simulink model "basebot_model_sampling"  (R2026a)
settings: Solver=ode45  StopTime=0.6  MaxStep=min(Ts/10,0.001)  RelTol=1e-6  AbsTol=1e-9
model workspace (MAT data in the model file):
  D = 1e-05
  J = 1e-05
  Kb = 0.01
  Kp = 0.05
  Kt = 0.01
  L = 0.001
  R = 1
  Ts = 0.001
  gear = 9.68
  referenceSpeed = 0.1
  stepTime = 0.2
  wheelRadius = 0.03
settings Model: Creator=michaeljohansen  LastModifiedBy=michaeljohansen

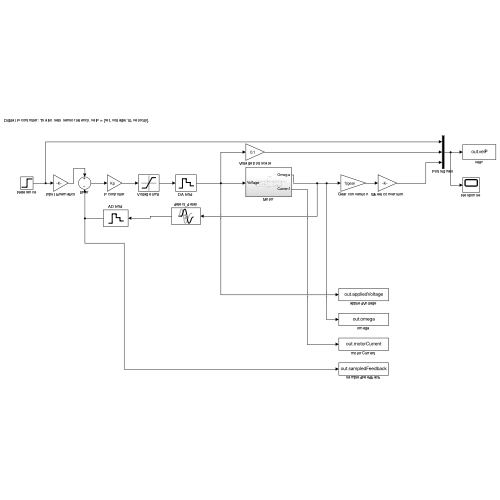
[thumbnail: Simulink's stored preview of the top-level diagram]
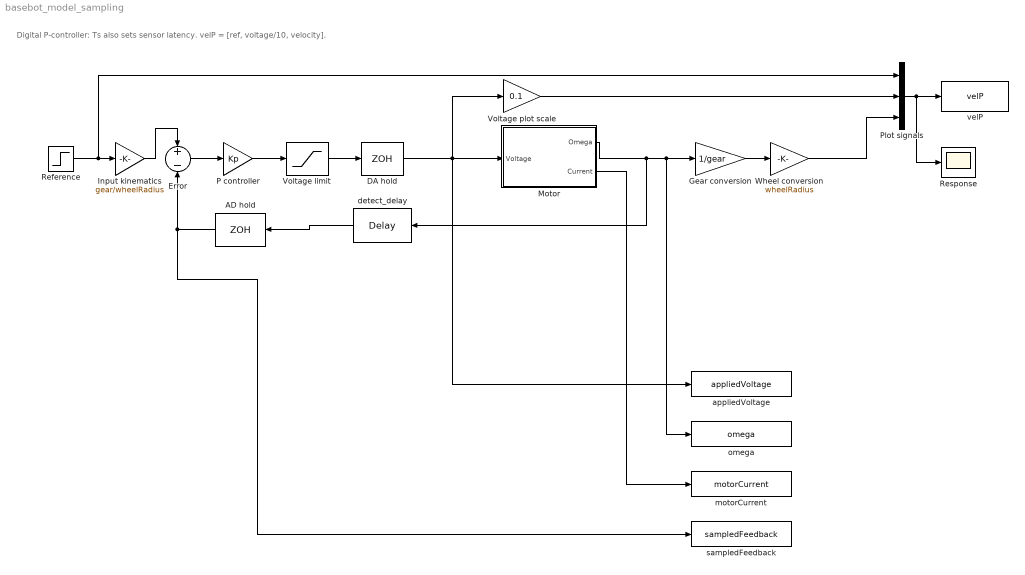
== system basebot_model_sampling ==
  note: Digital P-controller: Ts also sets sensor latency. velP = [ref, voltage/10, velocity].
  AD hold : ZeroOrderHold  SampleTime=Ts
  DA hold : ZeroOrderHold  SampleTime=Ts
  Error : Sum  Inputs=+-
  Gear conversion : Gain  Gain=1/gear
  Input kinematics : Gain  Gain=gear/wheelRadius
  Motor : Subsystem
  P controller : Gain  Gain=Kp
  Plot signals : Mux  Inputs=3
  Reference : Step  Time=stepTime  FinalValue=referenceSpeed  SampleTime=0
  Response : Scope
  Voltage limit : Saturate  UpperLimit=9  LowerLimit=-9
  Voltage plot scale : Gain  Gain=0.1
  Wheel conversion : Gain  Gain=wheelRadius
  appliedVoltage : ToWorkspace  VariableName=appliedVoltage  SaveFormat=Timeseries  SampleTime=-1
  detect_delay : TransportDelay  DelayTime=Ts
  motorCurrent : ToWorkspace  VariableName=motorCurrent  SaveFormat=Timeseries  SampleTime=-1
  omega : ToWorkspace  VariableName=omega  SaveFormat=Timeseries  SampleTime=-1
  sampledFeedback : ToWorkspace  VariableName=sampledFeedback  SaveFormat=Timeseries  SampleTime=-1
  velP : ToWorkspace  VariableName=velP  SaveFormat=Timeseries  SampleTime=-1
  wires:
  Reference/1 -> Input kinematics/1, Plot signals/1
  Input kinematics/1 -> Error/1
  Error/1 -> P controller/1
  P controller/1 -> Voltage limit/1
  Voltage limit/1 -> DA hold/1
  DA hold/1 -> Motor/1(Voltage), appliedVoltage/1, Voltage plot scale/1
  Motor/1(Omega) -> Gear conversion/1, omega/1, detect_delay/1
  detect_delay/1 -> AD hold/1
  AD hold/1 -> sampledFeedback/1, Error/2
  Gear conversion/1 -> Wheel conversion/1
  Voltage plot scale/1 -> Plot signals/2
  Wheel conversion/1 -> Plot signals/3
  Plot signals/1 -> velP/1, Response/1
  Motor/2(Current) -> motorCurrent/1

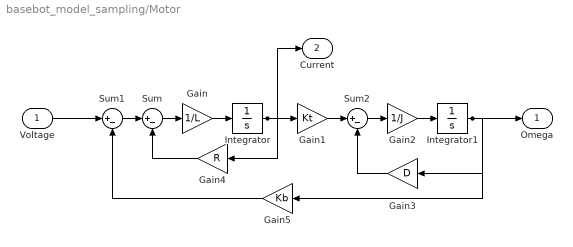
== system basebot_model_sampling/Motor ==
  Voltage : Inport
  Gain : Gain  Gain=1/L
  Gain1 : Gain  Gain=Kt
  Gain2 : Gain  Gain=1/J
  Gain3 : Gain  Gain=D
  Gain4 : Gain  Gain=R
  Gain5 : Gain  Gain=Kb
  Integrator : Integrator
  Integrator1 : Integrator
  Sum : Sum  Inputs=|+-
  Sum1 : Sum  Inputs=|+-
  Sum2 : Sum  Inputs=|+-
  Omega : Outport
  Current : Outport  Port=2
  wires:
  Voltage/1 -> Sum1/1
  Sum1/1 -> Sum/1
  Sum/1 -> Gain/1
  Gain/1 -> Integrator/1
  Integrator/1 -> Gain1/1, Gain4/1, Current/1
  Gain4/1 -> Sum/2
  Gain1/1 -> Sum2/1
  Sum2/1 -> Gain2/1
  Gain2/1 -> Integrator1/1
  Integrator1/1 -> Omega/1, Gain3/1, Gain5/1
  Gain3/1 -> Sum2/2
  Gain5/1 -> Sum1/2
